simulink subsystem "Cell_Module_with_Monitoring"  (R2022b)
settings: Solver=VariableStepAuto  StartTime=0.0  StopTime=10.0  RelTol=1e-3
settings Model: Creator=tshintai  LastModifiedBy=tshintai
settings DebuggingCC: UnconnectedInputMsg=warning  UnconnectedOutputMsg=warning  UnconnectedLineMsg=warning
settings ModelReferenceCC: EnableRefExpFcnMdlSchedulingChecks=on
settings RTWCC: DLArmComputeVersion=19.05

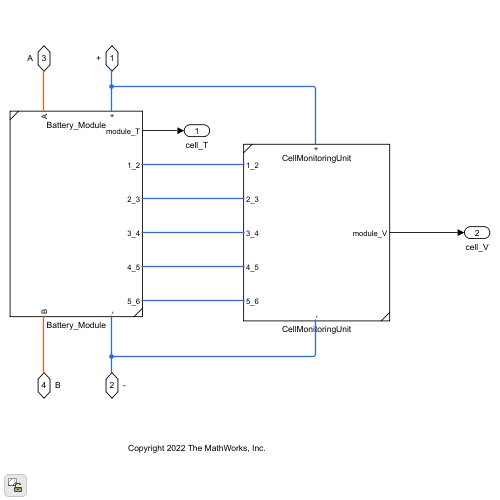
[thumbnail: Simulink's stored preview of the top-level diagram]
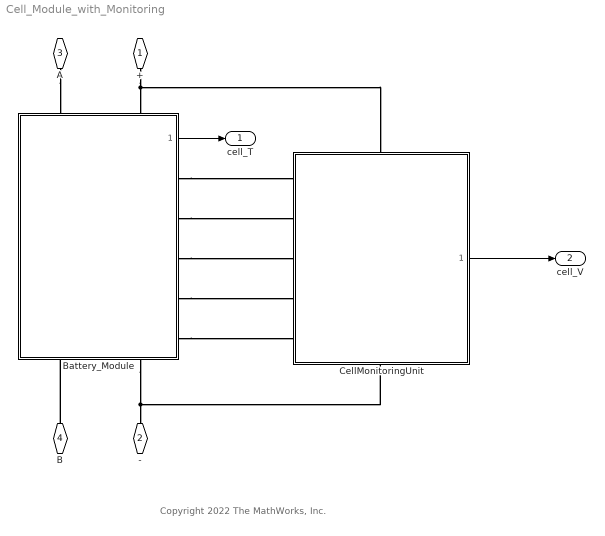
== system Cell_Module_with_Monitoring ==
  note: Copyright 2022 The MathWorks, Inc.
  Battery_Module : Subsystem  ReferencedSubsystem=Battery_Module
      settings: PortSchema="{\"entries\":[{\"content\":{\"sides\":[{\"content\":{\"connectorIds\":[]},\"type\":\"ConnectorPlacement.EquallySpacedRectSide\",\"uuid\":\"95cf6c26-c030-482e-89ff-aa008307b434\"},{\"content\":{\"connectorIds\":[\"Out1\",\"RConn2\",\"RConn3\",\"RConn4\",\"RConn5\",\"RConn6\"],\"side\":\"RIGHT\"},\"type\":\"ConnectorPlacement.EquallySpacedRectSide\",\"uuid\":\"a64fb354-bf29-4122-8ff8-3838c0310837\"},{\"content\":{\"connectorIds\":[\"RConn9\",\"RConn1\"],\"side\":\"TOP\"},\"type\":\"ConnectorPlacement.EquallySpacedRectSide\",\"uuid\":\"278f6031-fa48-4483-8ffe-09b62a90aff3\"},{\"content\":{\"connectorIds\":[\"RConn8\",\"RConn7\"],\"side\":\"BOTTOM\"},\"type\":\"ConnectorPlacement.EquallySpacedRectSide\",\"uuid\":\"209bfbc9-6393-4ca5-bc7c-dd76b491f783\"}]},\"type\":\"ConnectorPlacement.EquallySpacedConnector\",\"uuid\":\"04d6a708-eaaa-45ce-a76a-1b5d93280c81\"}],\"packageUris\":[\"http://schema.mathworks.com/mf0/Connector/R2020b\"],\"version\":\"1.0\"}"
  CellMonitoringUnit : Subsystem  ReferencedSubsystem=CellMonitoringUnit
      settings: PortSchema="{\"entries\":[{\"content\":{\"sides\":[{\"content\":{\"connectorIds\":[\"LConn2\",\"LConn3\",\"LConn4\",\"LConn5\",\"LConn6\"]},\"type\":\"ConnectorPlacement.EquallySpacedRectSide\",\"uuid\":\"25a6c8b6-584b-4e2f-a191-4ffafcc3e6b0\"},{\"content\":{\"connectorIds\":[\"Out1\"],\"side\":\"RIGHT\"},\"type\":\"ConnectorPlacement.EquallySpacedRectSide\",\"uuid\":\"29b90e12-133e-46d2-adfe-feb01948a60c\"},{\"content\":{\"connectorIds\":[\"LConn1\"],\"side\":\"TOP\"},\"type\":\"ConnectorPlacement.EquallySpacedRectSide\",\"uuid\":\"b11ea36c-d253-437f-932c-3bc80078a323\"},{\"content\":{\"connectorIds\":[\"LConn7\"],\"side\":\"BOTTOM\"},\"type\":\"ConnectorPlacement.EquallySpacedRectSide\",\"uuid\":\"f853e793-2eb9-4dab-9f11-7e5a5eea281f\"}]},\"type\":\"ConnectorPlacement.EquallySpacedConnector\",\"uuid\":\"e2b83178-8210-4e0d-af22-4a73fc58a6f2\"}],\"packageUris\":[\"http://schema.mathworks.com/mf0/Connector/R2020b\"],\"version\":\"1.0\"}"
  + : PMIOPort  Side=Left
  - : PMIOPort  Port=2  Side=Right
  A : PMIOPort  Port=3  Side=Left
  B : PMIOPort  Port=4  Side=Right
  cell_T : Outport
  cell_V : Outport  Port=2
  wires:
  CellMonitoringUnit/1 -> cell_V/1
  Battery_Module/1 -> cell_T/1
  connections:
  CellMonitoringUnit/LConn7 -- Battery_Module/RConn7 -- -/RConn1
  +/RConn1 -- Battery_Module/RConn1 -- CellMonitoringUnit/LConn1
  Battery_Module/RConn2 -- CellMonitoringUnit/LConn2
  Battery_Module/RConn5 -- CellMonitoringUnit/LConn5
  Battery_Module/RConn4 -- CellMonitoringUnit/LConn4
  Battery_Module/RConn6 -- CellMonitoringUnit/LConn6
  Battery_Module/RConn3 -- CellMonitoringUnit/LConn3
  A/RConn1 -- Battery_Module/RConn9
  B/RConn1 -- Battery_Module/RConn8
